simulink model "bloco_Modelo"  (R2015a)
settings: Solver=ode45  StartTime=0.0  StopTime=10.0  RelTol=1e-3
settings Model: Creator=YecidMoreno  LastModifiedBy=YecidMoreno

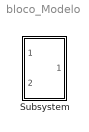
== system bloco_Modelo ==
  Subsystem : Subsystem

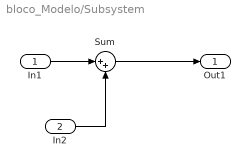
== system bloco_Modelo/Subsystem ==
  In1 : Inport
  In2 : Inport  Port=2
  Sum : Sum  Inputs=|++
  Out1 : Outport
  wires:
  Sum/1 -> Out1/1
  In1/1 -> Sum/1
  In2/1 -> Sum/2
